simulink model "RoboSoccerSim"  (R2022b)
settings: Solver=FixedStepAuto  StartTime=0.0  StopTime=inf  FixedStep=0.5  RelTol=1e-3
libraries: dspindex x20
settings Model: SimulationMode=accelerator  Creator=Wikian  LastModifiedBy=Sahil Gaurkar
settings ModelReferenceCC: EnableRefExpFcnMdlSchedulingChecks=on

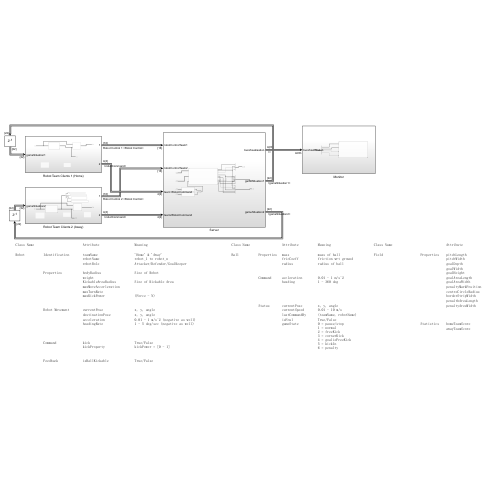
[thumbnail: Simulink's stored preview of the top-level diagram]
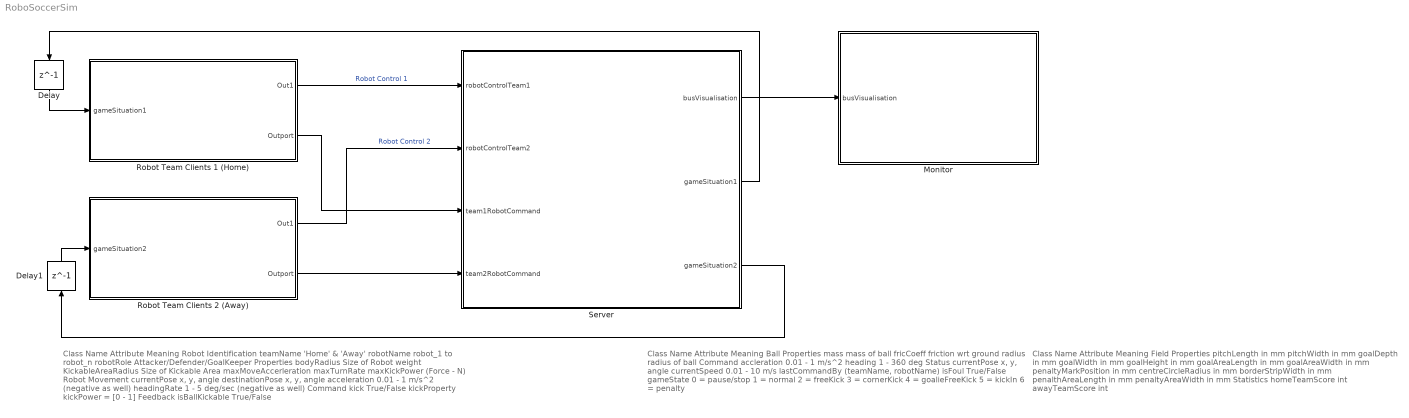
== system RoboSoccerSim ==
  note: Class Name
      |
      | Attribute
      | Meaning
      |
      | Field
      | Properties
      | pitchLength
      | in mm
      |
      | pitchWidth
      | in mm
      |
      | goalDepth
      | in mm
      |
      | goalWidth
      | in mm
      |
      | goalHeight
      | in mm
      |
      | goalAreaLength
      | in mm
      |
      | goalAreaWidth
      | in mm
      |
      | penaltyMarkPosition
      | in mm
      |
      | centreCircleRadius
      | in mm
      |
      | borderStripWidth
      | in mm
      |
      | penalthAreaLength
      | in mm
      |
      | penaltyAreaWidth
      | in mm
      |
      | Statistics
      | homeTeamScore
      | int
      |
      | awayTeamScore
      | int
  note: Class Name
      |
      | Attribute
      | Meaning
      |
      | Ball
      | Properties
      | mass
      | mass of ball
      |
      | fricCoeff
      | friction wrt ground
      |
      | radius
      | radius of ball
      |
      | Command
      | accleration
      | 0.01 - 1 m/s^2
      |
      | heading
      | 1 - 360 deg
      |
      | Status
      | currentPose
      | x, y, angle
      |
      | currentSpeed
      | 0.01 - 10 m/s
      |
      | lastCommandBy
      | (teamName, robotName)
      |
      | isFoul
      | True/False
      |
      | gameState
      | 0 = pause/stop
      | 1 = normal
      | 2 = freeKick
      | 3 = cornerKick
      | 4 = goalieFreeKick
      | 5 = kickIn
      | 6 = penalty
  note: Class Name
      |
      | Attribute
      | Meaning
      |
      | Robot
      | Identification
      | teamName
      | 'Home' & 'Away'
      |
      | robotName
      | robot_1 to robot_n
      |
      | robotRole
      | Attacker/Defender/GoalKeeper
      |
      | Properties
      | bodyRadius
      | Size of Robot
      |
      | weight
      |
      | KickableAreaRadius
      | Size of Kickable Area
      |
      | maxMoveAccerleration
      |
      | maxTurnRate
      |
      | maxKickPower
      | (Force - N)
      |
      | Robot Movement
      | currentPose
      | x, y, angle
      |
      | destinationPose
      | x, y, angle
      |
      | acceleration
      | 0.01 - 1 m/s^2 (negative as well)
      |
      | headingRate
      | 1 - 5 deg/sec (negative as well)
      |
      | Command
      | kick
      | True/False
      |
      | kickProperty
      | kickPower = [0 - 1]
      |
      | Feedback
      | isBallKickable
      | True/False
  Delay : Delay  DelayLength=1
  Delay1 : Delay  DelayLength=1
  Monitor : Subsystem
  Robot Team Clients 1 (Home) : Subsystem
  Robot Team Clients 2 (Away) : Subsystem
  Server : Subsystem
  wires:
  Robot Team Clients 1 (Home)/1(Out1) -> Server/1(robotControlTeam1)  "Robot Control 1"
  Robot Team Clients 2 (Away)/1(Out1) -> Server/2(robotControlTeam2)  "Robot Control 2"
  Server/1(busVisualisation) -> Monitor/1(busVisualisation)
  Server/3(gameSituation2) -> Delay1/1
  Server/2(gameSituation1) -> Delay/1
  Delay1/1 -> Robot Team Clients 2 (Away)/1(gameSituation2)
  Robot Team Clients 1 (Home)/2(Outport) -> Server/3(team1RobotCommand)
  Robot Team Clients 2 (Away)/2(Outport) -> Server/4(team2RobotCommand)
  Delay/1 -> Robot Team Clients 1 (Home)/1(gameSituation1)

== system RoboSoccerSim/Monitor ==
  busVisualisation : Inport
  Bus Selector : BusSelector  OutputSignals=robot coordinates and heading,ballCurrentPose,home team score,away team score
  Subsystem Reference : Subsystem  ReferencedSubsystem=Monitor_Subsystem
  wires:
  busVisualisation/1 -> Bus Selector/1
  Bus Selector/1 -> Subsystem Reference/1  "<robot coordinates and heading>"
  Bus Selector/2 -> Subsystem Reference/2  "<ballCurrentPose>"
  Bus Selector/3 -> Subsystem Reference/3  "<home team score>"
  Bus Selector/4 -> Subsystem Reference/4  "<away team score>"

== system RoboSoccerSim/Robot Team Clients 1 (Home) ==
  note: Signal: Robot Command
      |
      | 	robotDestinationPose
      | 	robotKick
      | 	robotKickProperty
  note: Signal: Game Situation
      | 	robotCurrentPose
      | 	ballGameState
      | 	ballCurrentPose
      | 	ballLastCommandBy
  gameSituation1 : Inport  OutDataTypeStr=Bus: gameSituation
  Robot Controllers : Subsystem
  Subsystem : Subsystem  ReferencedSubsystem=Guidance_Team1
  Out1 : Outport
  Outport : Outport  Port=2
  wires:
  gameSituation1/1 -> Robot Controllers/1(gameSituation), Subsystem/1  "gameSituation"
  Subsystem/1 -> Outport/1, Robot Controllers/2(robotCommand)  "robotCommand"
  Robot Controllers/1(Out1) -> Out1/1  "Robot Control"

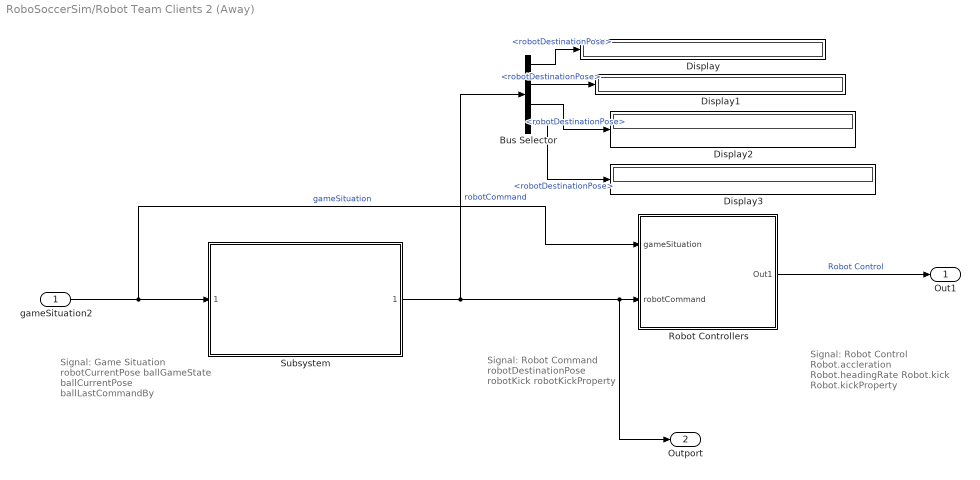
== system RoboSoccerSim/Robot Team Clients 2 (Away) ==
  note: Signal: Robot Control
      |
      | 	Robot.accleration
      | 	Robot.headingRate
      | 	Robot.kick
      | 	Robot.kickProperty
  note: Signal: Robot Command
      |
      | 	robotDestinationPose
      | 	robotKick
      | 	robotKickProperty
  note: Signal: Game Situation
      | 	robotCurrentPose
      | 	ballGameState
      | 	ballCurrentPose
      | 	ballLastCommandBy
  gameSituation2 : Inport  OutDataTypeStr=Bus:gameSituation
  Bus Selector : BusSelector  OutputSignals=robot1.robotDestinationPose,robot2.robotDestinationPose,robot3.robotDestinationPose,robot4.robotDestinationPose
  Display{,1..3} (4 alike) : Display
  Robot Controllers : Subsystem
  Subsystem : Subsystem  ReferencedSubsystem=Guidance_Team2
  Out1 : Outport
  Outport : Outport  Port=2
  wires:
  gameSituation2/1 -> Subsystem/1, Robot Controllers/1(gameSituation)  "gameSituation"
  Subsystem/1 -> Outport/1, Robot Controllers/2(robotCommand), Bus Selector/1  "robotCommand"
  Robot Controllers/1(Out1) -> Out1/1  "Robot Control"
  Bus Selector/1 -> Display/1  "<robotDestinationPose>"
  Bus Selector/2 -> Display1/1  "<robotDestinationPose>"
  Bus Selector/3 -> Display2/1  "<robotDestinationPose>"
  Bus Selector/4 -> Display3/1  "<robotDestinationPose>"

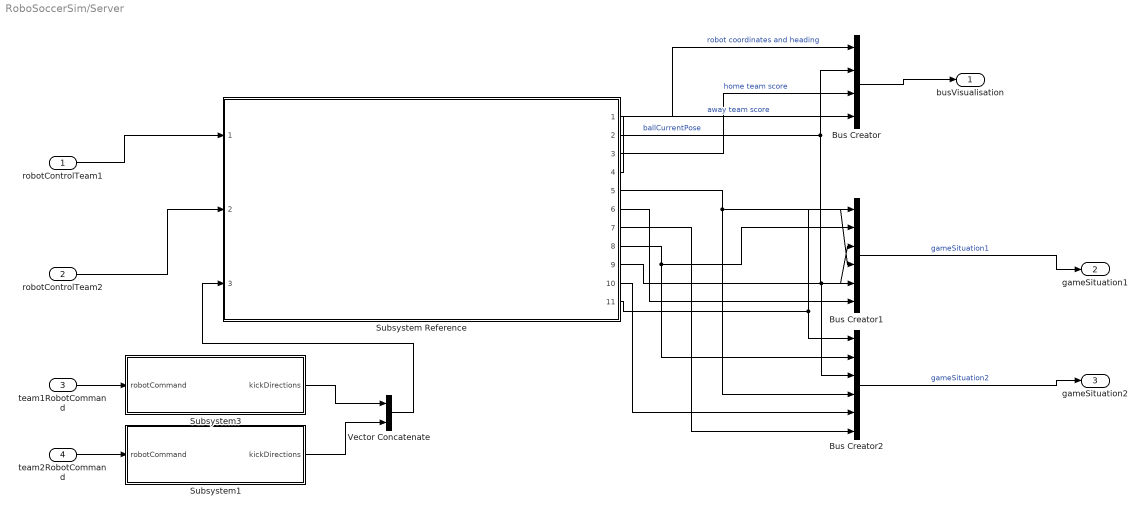
== system RoboSoccerSim/Server ==
  robotControlTeam1 : Inport
  robotControlTeam2 : Inport  Port=2
  team1RobotCommand : Inport  Port=3
  team2RobotCommand : Inport  Port=4
  Bus Creator : BusCreator  Inputs=4
  Bus Creator1 : BusCreator  Inputs=6  OutDataTypeStr=Bus: gameSituation
  Bus Creator2 : BusCreator  Inputs=6  OutDataTypeStr=Bus: gameSituation
  Subsystem Reference : Subsystem  ReferencedSubsystem=Server_sub
  Subsystem1 : Subsystem
  Subsystem3 : Subsystem
  Vector Concatenate : Concatenate
  busVisualisation : Outport
  gameSituation1 : Outport  Port=2
  gameSituation2 : Outport  Port=3
  wires:
  robotControlTeam2/1 -> Subsystem Reference/2
  robotControlTeam1/1 -> Subsystem Reference/1
  Subsystem Reference/1 -> Bus Creator/1  "robot coordinates and heading"
  Subsystem Reference/2 -> Bus Creator2/3, Bus Creator1/3, Bus Creator/2  "ballCurrentPose"
  Subsystem Reference/3 -> Bus Creator/3  "home team score"
  Subsystem Reference/4 -> Bus Creator/4  "away team score"
  Subsystem Reference/5 -> Bus Creator2/4, Bus Creator1/4
  Bus Creator/1 -> busVisualisation/1
  Subsystem Reference/6 -> Bus Creator1/6
  Subsystem Reference/8 -> Bus Creator2/2, Bus Creator1/2
  Subsystem Reference/9 -> Bus Creator1/5
  Subsystem Reference/11 -> Bus Creator2/1, Bus Creator1/1
  Bus Creator1/1 -> gameSituation1/1  "gameSituation1"
  Subsystem Reference/7 -> Bus Creator2/6
  Subsystem Reference/10 -> Bus Creator2/5
  Bus Creator2/1 -> gameSituation2/1  "gameSituation2"
  team1RobotCommand/1 -> Subsystem3/1(robotCommand)
  Subsystem3/1(kickDirections) -> Vector Concatenate/1
  team2RobotCommand/1 -> Subsystem1/1(robotCommand)
  Subsystem1/1(kickDirections) -> Vector Concatenate/2
  Vector Concatenate/1 -> Subsystem Reference/3

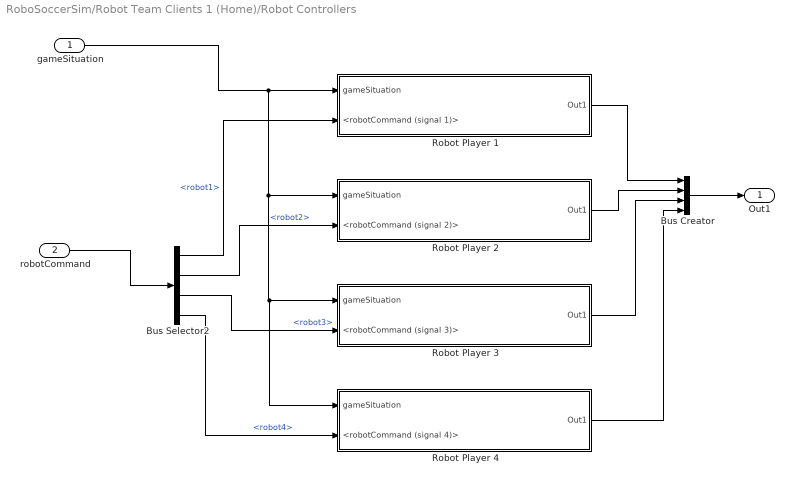
== system RoboSoccerSim/Robot Team Clients 1 (Home)/Robot Controllers ==
  gameSituation : Inport
  robotCommand : Inport  Port=2
  Bus Creator : BusCreator  Inputs=4
  Bus Selector2 : BusSelector  OutputSignals=robot1,robot2,robot3,robot4
  Robot Player 1 : Subsystem
  Robot Player 2 : Subsystem
  Robot Player 3 : Subsystem
  Robot Player 4 : Subsystem
  Out1 : Outport
  wires:
  Robot Player 1/1(Out1) -> Bus Creator/1
  Bus Creator/1 -> Out1/1
  robotCommand/1 -> Bus Selector2/1
  Bus Selector2/1 -> Robot Player 1/2(<robotCommand (signal 1)>)  "<robot1>"
  gameSituation/1 -> Robot Player 4/1(gameSituation), Robot Player 3/1(gameSituation), Robot Player 2/1(gameSituation), Robot Player 1/1(gameSituation)
  Bus Selector2/2 -> Robot Player 2/2(<robotCommand (signal 2)>)  "<robot2>"
  Bus Selector2/3 -> Robot Player 3/2(<robotCommand (signal 3)>)  "<robot3>"
  Robot Player 2/1(Out1) -> Bus Creator/2
  Robot Player 3/1(Out1) -> Bus Creator/3
  Robot Player 4/1(Out1) -> Bus Creator/4
  Bus Selector2/4 -> Robot Player 4/2(<robotCommand (signal 4)>)  "<robot4>"

== system RoboSoccerSim/Robot Team Clients 2 (Away)/Robot Controllers ==
  gameSituation : Inport
  robotCommand : Inport  Port=2
  Bus Creator : BusCreator  Inputs=4
  Bus Selector2 : BusSelector  OutputSignals=robot1,robot2,robot3,robot4
  Robot Player 1 : Subsystem
  Robot Player 2 : Subsystem
  Robot Player 3 : Subsystem
  Robot Player 4 : Subsystem
  Out1 : Outport
  wires:
  Robot Player 1/1(Out1) -> Bus Creator/1
  Bus Creator/1 -> Out1/1
  robotCommand/1 -> Bus Selector2/1
  Bus Selector2/1 -> Robot Player 1/2(<robotCommand (signal 1)>)  "<robot1>"
  gameSituation/1 -> Robot Player 4/1(gameSituation), Robot Player 3/1(gameSituation), Robot Player 2/1(gameSituation), Robot Player 1/1(gameSituation)
  Bus Selector2/2 -> Robot Player 2/2(<robotCommand (signal 2)>)  "<robot2>"
  Bus Selector2/3 -> Robot Player 3/2(<robotCommand (signal 3)>)  "<robot3>"
  Robot Player 2/1(Out1) -> Bus Creator/2
  Robot Player 3/1(Out1) -> Bus Creator/3
  Robot Player 4/1(Out1) -> Bus Creator/4
  Bus Selector2/4 -> Robot Player 4/2(<robotCommand (signal 4)>)  "<robot4>"

== system RoboSoccerSim/Server/Subsystem1 ==
  note: Signal: Robot Control
      |
      | 	Robot.accleration
      | 	Robot.headingRate
      | 	Robot.kick
      | 	Robot.kickProperty
  robotCommand : Inport
  Bus Selector2 : BusSelector  OutputSignals=robot1.robotDestinationPose,robot2.robotDestinationPose,robot3.robotDestinationPose,robot4.robotDestinationPose
  MATLAB Function : MATLAB Function  TreatAsAtomicUnit=on
  MATLAB Function1 : MATLAB Function  TreatAsAtomicUnit=on
  MATLAB Function2 : MATLAB Function  TreatAsAtomicUnit=on
  MATLAB Function3 : MATLAB Function  TreatAsAtomicUnit=on
  Vector Concatenate : Concatenate  NumInputs=4
  kickDirections : Outport
  wires:
  MATLAB Function/1(kickDirection) -> Vector Concatenate/1
  Vector Concatenate/1 -> kickDirections/1
  MATLAB Function1/1(kickDirection) -> Vector Concatenate/2
  robotCommand/1 -> Bus Selector2/1
  Bus Selector2/4 -> MATLAB Function3/1(destinationPose)  "<robotDestinationPose>"
  Bus Selector2/1 -> MATLAB Function/1(destinationPose)  "<robotDestinationPose>"
  MATLAB Function2/1(kickDirection) -> Vector Concatenate/3
  Bus Selector2/2 -> MATLAB Function1/1(destinationPose)  "<robotDestinationPose>"
  Bus Selector2/3 -> MATLAB Function2/1(destinationPose)  "<robotDestinationPose>"
  MATLAB Function3/1(kickDirection) -> Vector Concatenate/4

== system RoboSoccerSim/Server/Subsystem3 ==
  note: Signal: Robot Control
      |
      | 	Robot.accleration
      | 	Robot.headingRate
      | 	Robot.kick
      | 	Robot.kickProperty
  robotCommand : Inport
  Bus Selector2 : BusSelector  OutputSignals=robot1.robotDestinationPose,robot2.robotDestinationPose,robot3.robotDestinationPose,robot4.robotDestinationPose
  MATLAB Function : MATLAB Function  TreatAsAtomicUnit=on
  MATLAB Function1 : MATLAB Function  TreatAsAtomicUnit=on
  MATLAB Function2 : MATLAB Function  TreatAsAtomicUnit=on
  MATLAB Function3 : MATLAB Function  TreatAsAtomicUnit=on
  Vector Concatenate : Concatenate  NumInputs=4
  kickDirections : Outport
  wires:
  MATLAB Function/1(kickDirection) -> Vector Concatenate/1
  Vector Concatenate/1 -> kickDirections/1
  MATLAB Function1/1(kickDirection) -> Vector Concatenate/2
  robotCommand/1 -> Bus Selector2/1
  Bus Selector2/4 -> MATLAB Function3/1(destinationPose)  "<robotDestinationPose>"
  Bus Selector2/1 -> MATLAB Function/1(destinationPose)  "<robotDestinationPose>"
  MATLAB Function2/1(kickDirection) -> Vector Concatenate/3
  Bus Selector2/2 -> MATLAB Function1/1(destinationPose)  "<robotDestinationPose>"
  Bus Selector2/3 -> MATLAB Function2/1(destinationPose)  "<robotDestinationPose>"
  MATLAB Function3/1(kickDirection) -> Vector Concatenate/4

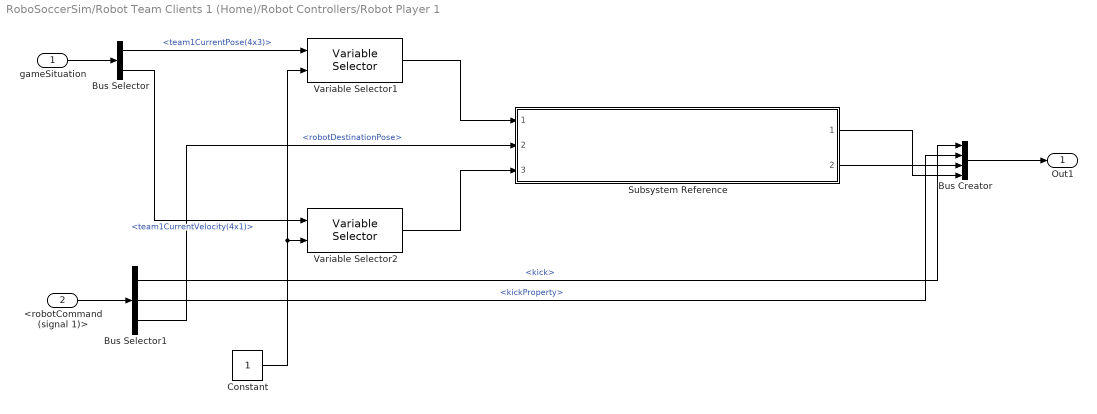
== system RoboSoccerSim/Robot Team Clients 1 (Home)/Robot Controllers/Robot Player 1 ==
  gameSituation : Inport
  <robotCommand (signal 1)> : Inport  Port=2
  Bus Creator : BusCreator  Inputs=4  OutDataTypeStr=Bus: robotControl
  Bus Selector : BusSelector  OutputSignals=team1CurrentPose(4x3),team1CurrentVelocity(4x1)
  Bus Selector1 : BusSelector  OutputSignals=kick,kickProperty,robotDestinationPose
  Constant : Constant
  Subsystem Reference : Subsystem  ReferencedSubsystem=Controller_Subsystem
  Variable Selector1 : dspindex/Variable Selector  NumInputs=1  rowsOrCols=Rows  IdxMode=Variable  Elements=[1 3]  ZerOneIdxMode=One-based  errmode=Clip Index  FillMode=on  FillValues=0
      settings: LibrarySourceBlock=|
      | dsphdlsupportsigmgmt/Variable
      | Selector
  Variable Selector2 : dspindex/Variable Selector  NumInputs=1  rowsOrCols=Rows  IdxMode=Variable  Elements=[1 3]  ZerOneIdxMode=One-based  errmode=Clip Index  FillMode=on  FillValues=0
      settings: LibrarySourceBlock=|
      | dsphdlsupportsigmgmt/Variable
      | Selector
  Out1 : Outport
  wires:
  Bus Selector1/3 -> Subsystem Reference/2  "<robotDestinationPose>"
  Constant/1 -> Variable Selector2/2, Variable Selector1/2
  Variable Selector1/1 -> Subsystem Reference/1
  Variable Selector2/1 -> Subsystem Reference/3
  gameSituation/1 -> Bus Selector/1
  Bus Selector/1 -> Variable Selector1/1  "<team1CurrentPose(4x3)>"
  Bus Selector/2 -> Variable Selector2/1  "<team1CurrentVelocity(4x1)>"
  <robotCommand (signal 1)>/1 -> Bus Selector1/1
  Bus Selector1/1 -> Bus Creator/1  "<kick>"
  Bus Selector1/2 -> Bus Creator/2  "<kickProperty>"
  Subsystem Reference/1 -> Bus Creator/4
  Subsystem Reference/2 -> Bus Creator/3
  Bus Creator/1 -> Out1/1

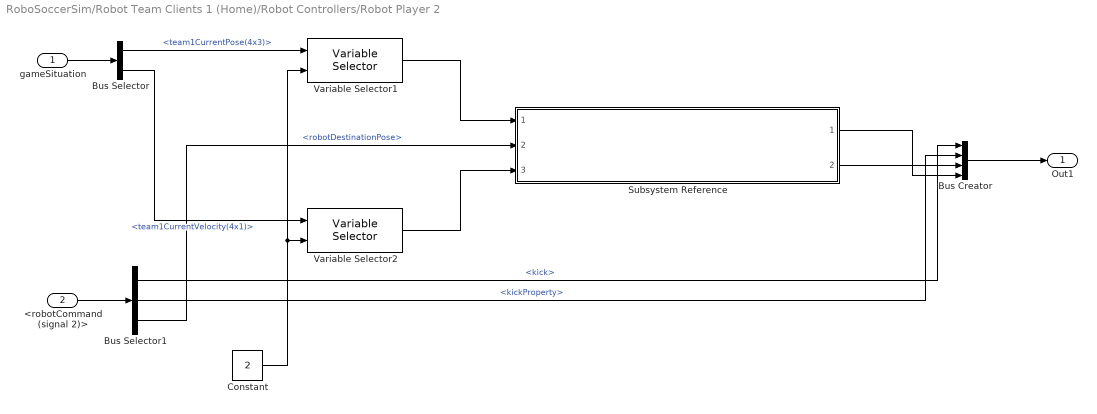
== system RoboSoccerSim/Robot Team Clients 1 (Home)/Robot Controllers/Robot Player 2 ==
  gameSituation : Inport
  <robotCommand (signal 2)> : Inport  Port=2
  Bus Creator : BusCreator  Inputs=4  OutDataTypeStr=Bus: robotControl
  Bus Selector : BusSelector  OutputSignals=team1CurrentPose(4x3),team1CurrentVelocity(4x1)
  Bus Selector1 : BusSelector  OutputSignals=kick,kickProperty,robotDestinationPose
  Constant : Constant  Value=2
  Subsystem Reference : Subsystem  ReferencedSubsystem=Controller_Subsystem
  Variable Selector1 : dspindex/Variable Selector  NumInputs=1  rowsOrCols=Rows  IdxMode=Variable  Elements=[1 3]  ZerOneIdxMode=One-based  errmode=Clip Index  FillMode=on  FillValues=0
      settings: LibrarySourceBlock=|
      | dsphdlsupportsigmgmt/Variable
      | Selector
  Variable Selector2 : dspindex/Variable Selector  NumInputs=1  rowsOrCols=Rows  IdxMode=Variable  Elements=[1 3]  ZerOneIdxMode=One-based  errmode=Clip Index  FillMode=on  FillValues=0
      settings: LibrarySourceBlock=|
      | dsphdlsupportsigmgmt/Variable
      | Selector
  Out1 : Outport
  wires:
  Bus Selector1/3 -> Subsystem Reference/2  "<robotDestinationPose>"
  Constant/1 -> Variable Selector2/2, Variable Selector1/2
  Variable Selector1/1 -> Subsystem Reference/1
  Variable Selector2/1 -> Subsystem Reference/3
  gameSituation/1 -> Bus Selector/1
  Bus Selector/1 -> Variable Selector1/1  "<team1CurrentPose(4x3)>"
  Bus Selector/2 -> Variable Selector2/1  "<team1CurrentVelocity(4x1)>"
  <robotCommand (signal 2)>/1 -> Bus Selector1/1
  Bus Selector1/1 -> Bus Creator/1  "<kick>"
  Bus Selector1/2 -> Bus Creator/2  "<kickProperty>"
  Subsystem Reference/1 -> Bus Creator/4
  Subsystem Reference/2 -> Bus Creator/3
  Bus Creator/1 -> Out1/1

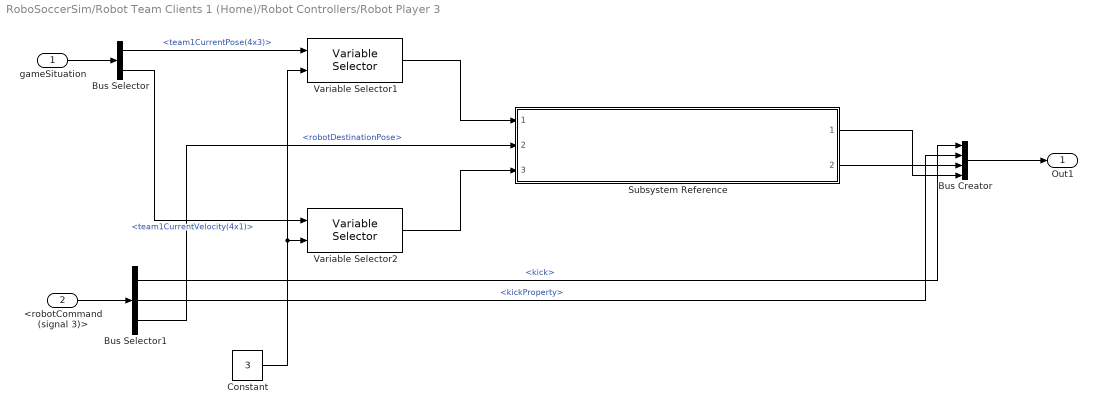
== system RoboSoccerSim/Robot Team Clients 1 (Home)/Robot Controllers/Robot Player 3 ==
  gameSituation : Inport
  <robotCommand (signal 3)> : Inport  Port=2
  Bus Creator : BusCreator  Inputs=4  OutDataTypeStr=Bus: robotControl
  Bus Selector : BusSelector  OutputSignals=team1CurrentPose(4x3),team1CurrentVelocity(4x1)
  Bus Selector1 : BusSelector  OutputSignals=kick,kickProperty,robotDestinationPose
  Constant : Constant  Value=3
  Subsystem Reference : Subsystem  ReferencedSubsystem=Controller_Subsystem
  Variable Selector1 : dspindex/Variable Selector  NumInputs=1  rowsOrCols=Rows  IdxMode=Variable  Elements=[1 3]  ZerOneIdxMode=One-based  errmode=Clip Index  FillMode=on  FillValues=0
      settings: LibrarySourceBlock=|
      | dsphdlsupportsigmgmt/Variable
      | Selector
  Variable Selector2 : dspindex/Variable Selector  NumInputs=1  rowsOrCols=Rows  IdxMode=Variable  Elements=[1 3]  ZerOneIdxMode=One-based  errmode=Clip Index  FillMode=on  FillValues=0
      settings: LibrarySourceBlock=|
      | dsphdlsupportsigmgmt/Variable
      | Selector
  Out1 : Outport
  wires:
  Bus Selector1/3 -> Subsystem Reference/2  "<robotDestinationPose>"
  Constant/1 -> Variable Selector2/2, Variable Selector1/2
  Variable Selector1/1 -> Subsystem Reference/1
  Variable Selector2/1 -> Subsystem Reference/3
  gameSituation/1 -> Bus Selector/1
  Bus Selector/1 -> Variable Selector1/1  "<team1CurrentPose(4x3)>"
  Bus Selector/2 -> Variable Selector2/1  "<team1CurrentVelocity(4x1)>"
  <robotCommand (signal 3)>/1 -> Bus Selector1/1
  Bus Selector1/1 -> Bus Creator/1  "<kick>"
  Bus Selector1/2 -> Bus Creator/2  "<kickProperty>"
  Subsystem Reference/1 -> Bus Creator/4
  Subsystem Reference/2 -> Bus Creator/3
  Bus Creator/1 -> Out1/1

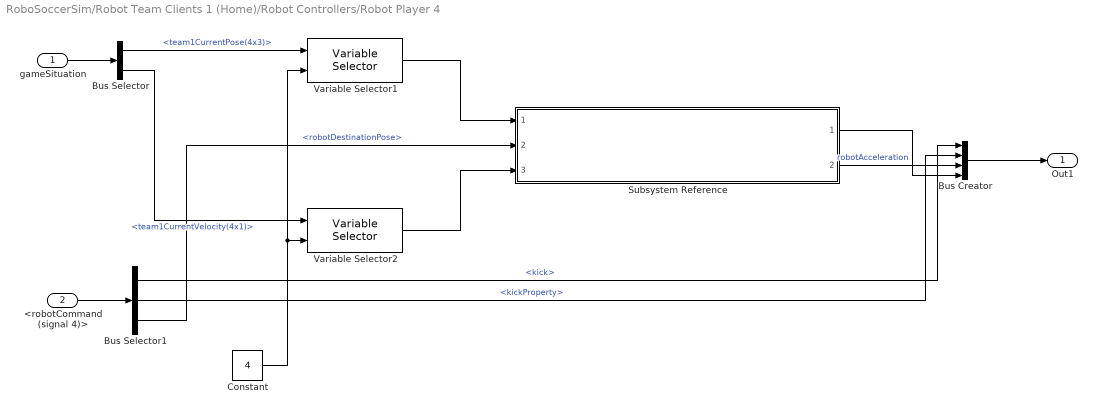
== system RoboSoccerSim/Robot Team Clients 1 (Home)/Robot Controllers/Robot Player 4 ==
  gameSituation : Inport
  <robotCommand (signal 4)> : Inport  Port=2
  Bus Creator : BusCreator  Inputs=4  OutDataTypeStr=Bus: robotControl
  Bus Selector : BusSelector  OutputSignals=team1CurrentPose(4x3),team1CurrentVelocity(4x1)
  Bus Selector1 : BusSelector  OutputSignals=kick,kickProperty,robotDestinationPose
  Constant : Constant  Value=4
  Subsystem Reference : Subsystem  ReferencedSubsystem=Controller_Subsystem
  Variable Selector1 : dspindex/Variable Selector  NumInputs=1  rowsOrCols=Rows  IdxMode=Variable  Elements=[1 3]  ZerOneIdxMode=One-based  errmode=Clip Index  FillMode=on  FillValues=0
      settings: LibrarySourceBlock=|
      | dsphdlsupportsigmgmt/Variable
      | Selector
  Variable Selector2 : dspindex/Variable Selector  NumInputs=1  rowsOrCols=Rows  IdxMode=Variable  Elements=[1 3]  ZerOneIdxMode=One-based  errmode=Clip Index  FillMode=on  FillValues=0
      settings: LibrarySourceBlock=|
      | dsphdlsupportsigmgmt/Variable
      | Selector
  Out1 : Outport
  wires:
  Bus Selector1/3 -> Subsystem Reference/2  "<robotDestinationPose>"
  Constant/1 -> Variable Selector2/2, Variable Selector1/2
  Variable Selector1/1 -> Subsystem Reference/1
  Variable Selector2/1 -> Subsystem Reference/3
  gameSituation/1 -> Bus Selector/1
  Bus Selector/1 -> Variable Selector1/1  "<team1CurrentPose(4x3)>"
  Bus Selector/2 -> Variable Selector2/1  "<team1CurrentVelocity(4x1)>"
  <robotCommand (signal 4)>/1 -> Bus Selector1/1
  Bus Selector1/1 -> Bus Creator/1  "<kick>"
  Bus Selector1/2 -> Bus Creator/2  "<kickProperty>"
  Subsystem Reference/1 -> Bus Creator/4
  Subsystem Reference/2 -> Bus Creator/3  "robotAcceleration"
  Bus Creator/1 -> Out1/1

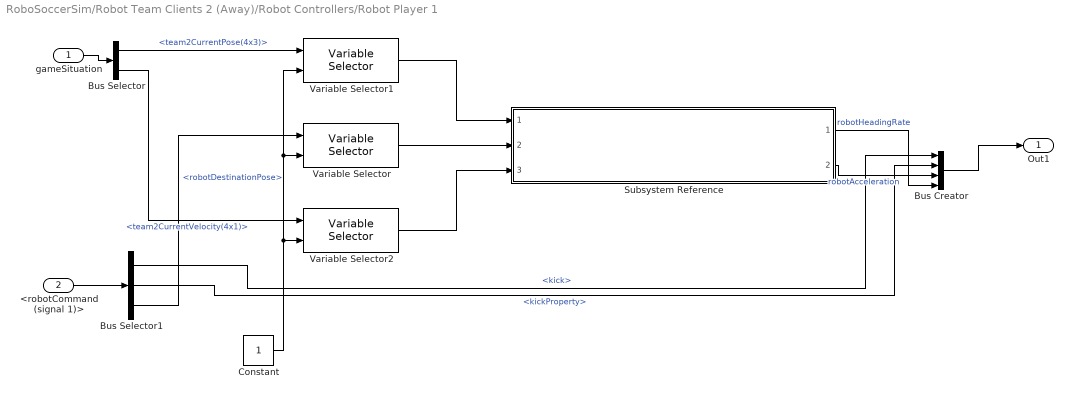
== system RoboSoccerSim/Robot Team Clients 2 (Away)/Robot Controllers/Robot Player 1 ==
  gameSituation : Inport
  <robotCommand (signal 1)> : Inport  Port=2
  Bus Creator : BusCreator  Inputs=4  OutDataTypeStr=Bus: robotControl
  Bus Selector : BusSelector  OutputSignals=team2CurrentPose(4x3),team2CurrentVelocity(4x1)
  Bus Selector1 : BusSelector  OutputSignals=kick,kickProperty,robotDestinationPose
  Constant : Constant
  Subsystem Reference : Subsystem  ReferencedSubsystem=Controller_Subsystem
  Variable Selector : dspindex/Variable Selector  NumInputs=1  rowsOrCols=Rows  IdxMode=Variable  Elements=[1 3]  ZerOneIdxMode=One-based  errmode=Clip Index  FillMode=on  FillValues=0
      settings: LibrarySourceBlock=|
      | dsphdlsupportsigmgmt/Variable
      | Selector
  Variable Selector1 : dspindex/Variable Selector  NumInputs=1  rowsOrCols=Rows  IdxMode=Variable  Elements=[1 3]  ZerOneIdxMode=One-based  errmode=Clip Index  FillMode=on  FillValues=0
      settings: LibrarySourceBlock=|
      | dsphdlsupportsigmgmt/Variable
      | Selector
  Variable Selector2 : dspindex/Variable Selector  NumInputs=1  rowsOrCols=Rows  IdxMode=Variable  Elements=[1 3]  ZerOneIdxMode=One-based  errmode=Clip Index  FillMode=on  FillValues=0
      settings: LibrarySourceBlock=|
      | dsphdlsupportsigmgmt/Variable
      | Selector
  Out1 : Outport
  wires:
  Bus Selector1/3 -> Variable Selector/1  "<robotDestinationPose>"
  Variable Selector/1 -> Subsystem Reference/2
  Constant/1 -> Variable Selector2/2, Variable Selector1/2, Variable Selector/2
  Variable Selector1/1 -> Subsystem Reference/1
  Variable Selector2/1 -> Subsystem Reference/3
  gameSituation/1 -> Bus Selector/1
  Bus Selector/2 -> Variable Selector2/1  "<team2CurrentVelocity(4x1)>"
  <robotCommand (signal 1)>/1 -> Bus Selector1/1
  Bus Selector1/1 -> Bus Creator/1  "<kick>"
  Bus Selector1/2 -> Bus Creator/2  "<kickProperty>"
  Subsystem Reference/1 -> Bus Creator/4  "robotHeadingRate"
  Subsystem Reference/2 -> Bus Creator/3  "robotAcceleration"
  Bus Creator/1 -> Out1/1
  Bus Selector/1 -> Variable Selector1/1  "<team2CurrentPose(4x3)>"

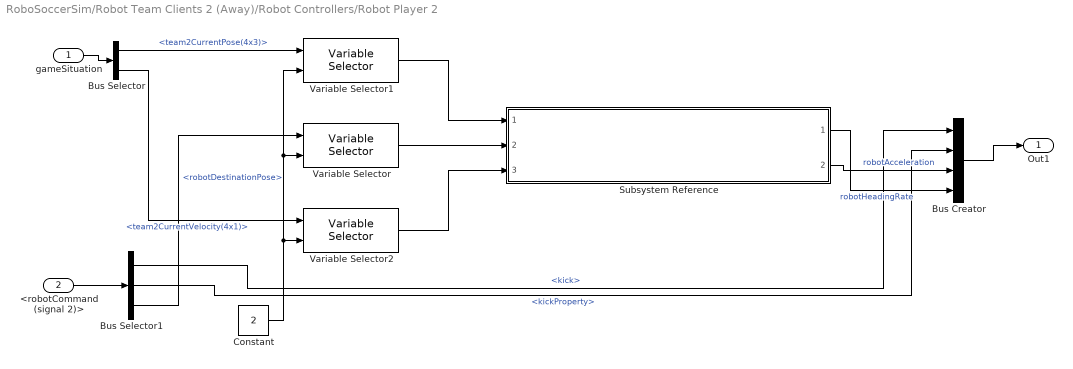
== system RoboSoccerSim/Robot Team Clients 2 (Away)/Robot Controllers/Robot Player 2 ==
  gameSituation : Inport
  <robotCommand (signal 2)> : Inport  Port=2
  Bus Creator : BusCreator  Inputs=4  OutDataTypeStr=Bus: robotControl
  Bus Selector : BusSelector  OutputSignals=team2CurrentPose(4x3),team2CurrentVelocity(4x1)
  Bus Selector1 : BusSelector  OutputSignals=kick,kickProperty,robotDestinationPose
  Constant : Constant  Value=2
  Subsystem Reference : Subsystem  ReferencedSubsystem=Controller_Subsystem
  Variable Selector : dspindex/Variable Selector  NumInputs=1  rowsOrCols=Rows  IdxMode=Variable  Elements=[1 3]  ZerOneIdxMode=One-based  errmode=Clip Index  FillMode=on  FillValues=0
      settings: LibrarySourceBlock=|
      | dsphdlsupportsigmgmt/Variable
      | Selector
  Variable Selector1 : dspindex/Variable Selector  NumInputs=1  rowsOrCols=Rows  IdxMode=Variable  Elements=[1 3]  ZerOneIdxMode=One-based  errmode=Clip Index  FillMode=on  FillValues=0
      settings: LibrarySourceBlock=|
      | dsphdlsupportsigmgmt/Variable
      | Selector
  Variable Selector2 : dspindex/Variable Selector  NumInputs=1  rowsOrCols=Rows  IdxMode=Variable  Elements=[1 3]  ZerOneIdxMode=One-based  errmode=Clip Index  FillMode=on  FillValues=0
      settings: LibrarySourceBlock=|
      | dsphdlsupportsigmgmt/Variable
      | Selector
  Out1 : Outport
  wires:
  Bus Selector1/3 -> Variable Selector/1  "<robotDestinationPose>"
  Variable Selector/1 -> Subsystem Reference/2
  Constant/1 -> Variable Selector2/2, Variable Selector1/2, Variable Selector/2
  Variable Selector1/1 -> Subsystem Reference/1
  Variable Selector2/1 -> Subsystem Reference/3
  gameSituation/1 -> Bus Selector/1
  Bus Selector/2 -> Variable Selector2/1  "<team2CurrentVelocity(4x1)>"
  <robotCommand (signal 2)>/1 -> Bus Selector1/1
  Bus Selector1/1 -> Bus Creator/1  "<kick>"
  Bus Selector1/2 -> Bus Creator/2  "<kickProperty>"
  Subsystem Reference/1 -> Bus Creator/4  "robotHeadingRate"
  Subsystem Reference/2 -> Bus Creator/3  "robotAcceleration"
  Bus Creator/1 -> Out1/1
  Bus Selector/1 -> Variable Selector1/1  "<team2CurrentPose(4x3)>"

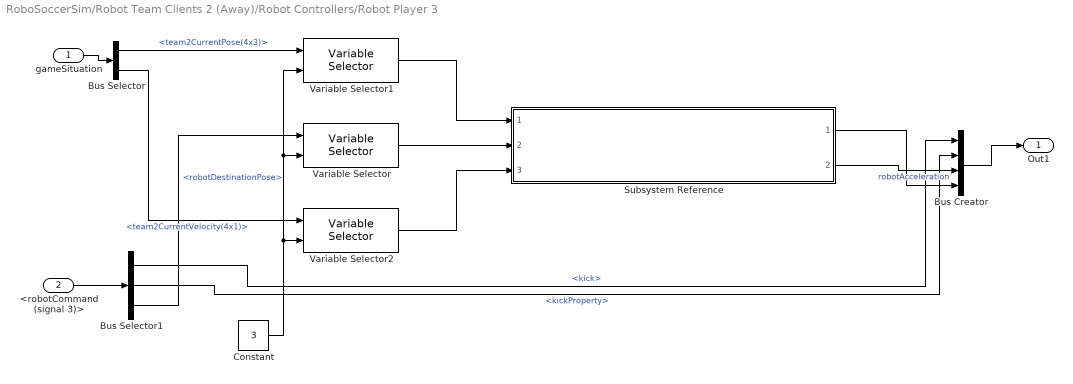
== system RoboSoccerSim/Robot Team Clients 2 (Away)/Robot Controllers/Robot Player 3 ==
  gameSituation : Inport
  <robotCommand (signal 3)> : Inport  Port=2
  Bus Creator : BusCreator  Inputs=4  OutDataTypeStr=Bus: robotControl
  Bus Selector : BusSelector  OutputSignals=team2CurrentPose(4x3),team2CurrentVelocity(4x1)
  Bus Selector1 : BusSelector  OutputSignals=kick,kickProperty,robotDestinationPose
  Constant : Constant  Value=3
  Subsystem Reference : Subsystem  ReferencedSubsystem=Controller_Subsystem
  Variable Selector : dspindex/Variable Selector  NumInputs=1  rowsOrCols=Rows  IdxMode=Variable  Elements=[1 3]  ZerOneIdxMode=One-based  errmode=Clip Index  FillMode=on  FillValues=0
      settings: LibrarySourceBlock=|
      | dsphdlsupportsigmgmt/Variable
      | Selector
  Variable Selector1 : dspindex/Variable Selector  NumInputs=1  rowsOrCols=Rows  IdxMode=Variable  Elements=[1 3]  ZerOneIdxMode=One-based  errmode=Clip Index  FillMode=on  FillValues=0
      settings: LibrarySourceBlock=|
      | dsphdlsupportsigmgmt/Variable
      | Selector
  Variable Selector2 : dspindex/Variable Selector  NumInputs=1  rowsOrCols=Rows  IdxMode=Variable  Elements=[1 3]  ZerOneIdxMode=One-based  errmode=Clip Index  FillMode=on  FillValues=0
      settings: LibrarySourceBlock=|
      | dsphdlsupportsigmgmt/Variable
      | Selector
  Out1 : Outport
  wires:
  Bus Selector1/3 -> Variable Selector/1  "<robotDestinationPose>"
  Variable Selector/1 -> Subsystem Reference/2
  Constant/1 -> Variable Selector2/2, Variable Selector1/2, Variable Selector/2
  Variable Selector1/1 -> Subsystem Reference/1
  Variable Selector2/1 -> Subsystem Reference/3
  gameSituation/1 -> Bus Selector/1
  Bus Selector/2 -> Variable Selector2/1  "<team2CurrentVelocity(4x1)>"
  <robotCommand (signal 3)>/1 -> Bus Selector1/1
  Bus Selector1/1 -> Bus Creator/1  "<kick>"
  Bus Selector1/2 -> Bus Creator/2  "<kickProperty>"
  Subsystem Reference/1 -> Bus Creator/4
  Subsystem Reference/2 -> Bus Creator/3  "robotAcceleration"
  Bus Creator/1 -> Out1/1
  Bus Selector/1 -> Variable Selector1/1  "<team2CurrentPose(4x3)>"

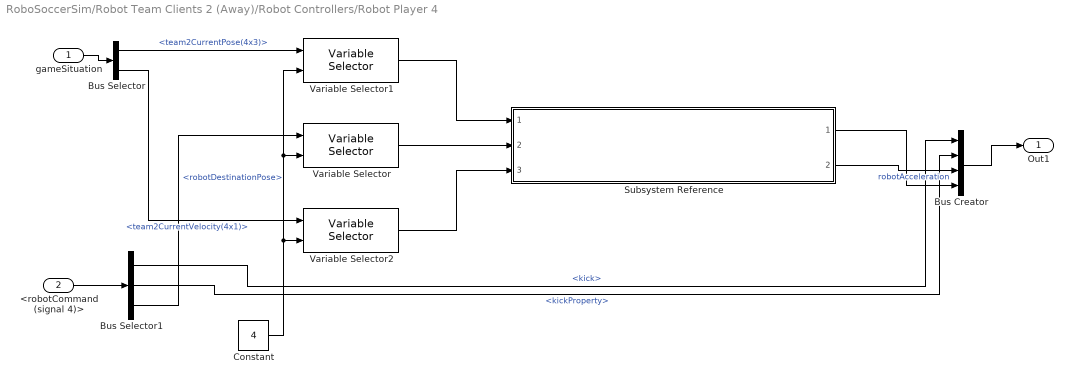
== system RoboSoccerSim/Robot Team Clients 2 (Away)/Robot Controllers/Robot Player 4 ==
  gameSituation : Inport
  <robotCommand (signal 4)> : Inport  Port=2
  Bus Creator : BusCreator  Inputs=4  OutDataTypeStr=Bus: robotControl
  Bus Selector : BusSelector  OutputSignals=team2CurrentPose(4x3),team2CurrentVelocity(4x1)
  Bus Selector1 : BusSelector  OutputSignals=kick,kickProperty,robotDestinationPose
  Constant : Constant  Value=4
  Subsystem Reference : Subsystem  ReferencedSubsystem=Controller_Subsystem
  Variable Selector : dspindex/Variable Selector  NumInputs=1  rowsOrCols=Rows  IdxMode=Variable  Elements=[1 3]  ZerOneIdxMode=One-based  errmode=Clip Index  FillMode=on  FillValues=0
      settings: LibrarySourceBlock=|
      | dsphdlsupportsigmgmt/Variable
      | Selector
  Variable Selector1 : dspindex/Variable Selector  NumInputs=1  rowsOrCols=Rows  IdxMode=Variable  Elements=[1 3]  ZerOneIdxMode=One-based  errmode=Clip Index  FillMode=on  FillValues=0
      settings: LibrarySourceBlock=|
      | dsphdlsupportsigmgmt/Variable
      | Selector
  Variable Selector2 : dspindex/Variable Selector  NumInputs=1  rowsOrCols=Rows  IdxMode=Variable  Elements=[1 3]  ZerOneIdxMode=One-based  errmode=Clip Index  FillMode=on  FillValues=0
      settings: LibrarySourceBlock=|
      | dsphdlsupportsigmgmt/Variable
      | Selector
  Out1 : Outport
  wires:
  Bus Selector1/3 -> Variable Selector/1  "<robotDestinationPose>"
  Variable Selector/1 -> Subsystem Reference/2
  Constant/1 -> Variable Selector2/2, Variable Selector1/2, Variable Selector/2
  Variable Selector1/1 -> Subsystem Reference/1
  Variable Selector2/1 -> Subsystem Reference/3
  gameSituation/1 -> Bus Selector/1
  Bus Selector/2 -> Variable Selector2/1  "<team2CurrentVelocity(4x1)>"
  <robotCommand (signal 4)>/1 -> Bus Selector1/1
  Bus Selector1/1 -> Bus Creator/1  "<kick>"
  Bus Selector1/2 -> Bus Creator/2  "<kickProperty>"
  Subsystem Reference/1 -> Bus Creator/4
  Subsystem Reference/2 -> Bus Creator/3  "robotAcceleration"
  Bus Creator/1 -> Out1/1
  Bus Selector/1 -> Variable Selector1/1  "<team2CurrentPose(4x3)>"

== matlab function RoboSoccerSim/Server/Subsystem3/MATLAB Function ==
  data: kickDirection output; destinationPose input
function kickDirection  = fcn(destinationPose)

kickDirection = destinationPose(3);

end

== matlab function RoboSoccerSim/Server/Subsystem3/MATLAB Function1 ==
  data: kickDirection output; destinationPose input
function kickDirection  = fcn(destinationPose)

kickDirection = destinationPose(3);

end

== matlab function RoboSoccerSim/Server/Subsystem3/MATLAB Function2 ==
  data: kickDirection output; destinationPose input
function kickDirection  = fcn(destinationPose)

kickDirection = destinationPose(3);

end

== matlab function RoboSoccerSim/Server/Subsystem3/MATLAB Function3 ==
  data: kickDirection output; destinationPose input
function kickDirection  = fcn(destinationPose)

kickDirection = destinationPose(3);

end

== matlab function RoboSoccerSim/Server/Subsystem1/MATLAB Function ==
  data: kickDirection output; destinationPose input
function kickDirection  = fcn(destinationPose)

kickDirection = destinationPose(3);

end

== matlab function RoboSoccerSim/Server/Subsystem1/MATLAB Function1 ==
  data: kickDirection output; destinationPose input
function kickDirection  = fcn(destinationPose)

kickDirection = destinationPose(3);

end

== matlab function RoboSoccerSim/Server/Subsystem1/MATLAB Function2 ==
  data: kickDirection output; destinationPose input
function kickDirection  = fcn(destinationPose)

kickDirection = destinationPose(3);

end

== matlab function RoboSoccerSim/Server/Subsystem1/MATLAB Function3 ==
  data: kickDirection output; destinationPose input
function kickDirection  = fcn(destinationPose)

kickDirection = destinationPose(3);

end
